simulink model "foc_decoupling_test"  (R2015a)
settings: Solver=ode45  StartTime=0.0  StopTime=0.01  RelTol=1e-3
libraries: simulink x2
settings Model: Creator=user  LastModifiedBy=user

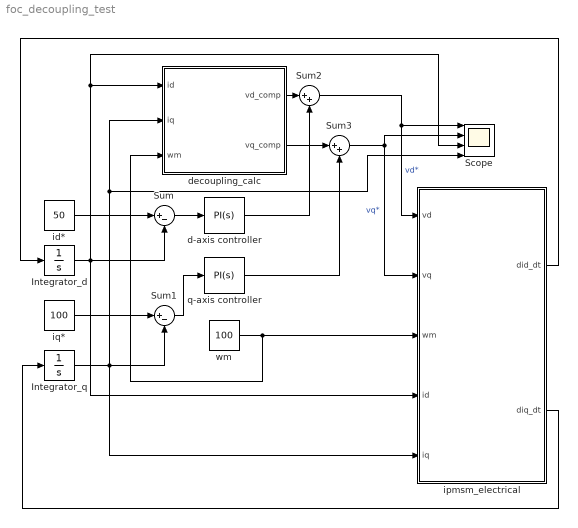
== system foc_decoupling_test ==
  Integrator_d : Integrator
  Integrator_q : Integrator
  Scope : Scope  NumInputPorts=4
      settings: YMin=-5~-5~-5~-5  YMax=5~5~5~5  SaveName=ScopeData2
  Sum : Sum  Inputs=|+-
  Sum1 : Sum  Inputs=|+-
  Sum2 : Sum  Inputs=|++
  Sum3 : Sum  Inputs=|++
  d-axis controller : simulink/Continuous/PID Controller  Controller=PI  TimeDomain=Continuous-time  SampleTime=-1  IntegratorMethod=Forward Euler  FilterMethod=Forward Euler  Form=Parallel  UseFilter=on  ControllerParametersSource=internal  P=0.2827  I=16.6504  D=0  N=100  InitialConditionSource=internal  InitialConditionForIntegrator=0  InitialConditionForFilter=0  ExternalReset=none  LimitOutput=off  UpperSaturationLimit=inf  LowerSaturationLimit=-inf  LinearizeAsGain=on  AntiWindupMode=none  Kb=1  TrackingMode=off  Kt=1  PParamMin=[]  PParamMax=[]  IParamMin=[]  IParamMax=[]  DParamMin=[]  DParamMax=[]  NParamMin=[]  NParamMax=[]  KbParamMin=[]  KbParamMax=[]  KtParamMin=[]  KtParamMax=[]  POutMin=[]  POutMax=[]  IOutMin=[]  IOutMax=[]  DOutMin=[]  DOutMax=[]  NOutMin=[]  NOutMax=[]  KbOutMin=[]  KbOutMax=[]  KtOutMin=[]  KtOutMax=[]  IntegratorOutMin=[]  IntegratorOutMax=[]  FilterOutMin=[]  FilterOutMax=[]  SumOutMin=[]  SumOutMax=[]  SumI1OutMin=[]  SumI1OutMax=[]  SumI2OutMin=[]  SumI2OutMax=[]  SumI3OutMin=[]  SumI3OutMax=[]  SumDOutMin=[]  SumDOutMax=[]  SaturationOutMin=[]  SaturationOutMax=[]  IntegratorContinuousStateAttributes=''  IntegratorStateMustResolveToSignalObject=off  IntegratorRTWStateStorageClass=Auto  FilterContinuousStateAttributes=''  FilterStateMustResolveToSignalObject=off  FilterRTWStateStorageClass=Auto  DifferentiatorICPrevScaledInput=0  DifferentiatorOutMin=[]  DifferentiatorOutMax=[]
  decoupling_calc : MATLAB Function  TreatAsAtomicUnit=on
  id* : Constant  Value=50
  ipmsm_electrical : MATLAB Function  TreatAsAtomicUnit=on
  iq* : Constant  Value=100
  q-axis controller : simulink/Continuous/PID Controller  Controller=PI  TimeDomain=Continuous-time  SampleTime=-1  IntegratorMethod=Forward Euler  FilterMethod=Forward Euler  Form=Parallel  UseFilter=on  ControllerParametersSource=internal  P=0.8011  I=16.6504  D=0  N=100  InitialConditionSource=internal  InitialConditionForIntegrator=0  InitialConditionForFilter=0  ExternalReset=none  LimitOutput=off  UpperSaturationLimit=inf  LowerSaturationLimit=-inf  LinearizeAsGain=on  AntiWindupMode=none  Kb=1  TrackingMode=off  Kt=1  PParamMin=[]  PParamMax=[]  IParamMin=[]  IParamMax=[]  DParamMin=[]  DParamMax=[]  NParamMin=[]  NParamMax=[]  KbParamMin=[]  KbParamMax=[]  KtParamMin=[]  KtParamMax=[]  POutMin=[]  POutMax=[]  IOutMin=[]  IOutMax=[]  DOutMin=[]  DOutMax=[]  NOutMin=[]  NOutMax=[]  KbOutMin=[]  KbOutMax=[]  KtOutMin=[]  KtOutMax=[]  IntegratorOutMin=[]  IntegratorOutMax=[]  FilterOutMin=[]  FilterOutMax=[]  SumOutMin=[]  SumOutMax=[]  SumI1OutMin=[]  SumI1OutMax=[]  SumI2OutMin=[]  SumI2OutMax=[]  SumI3OutMin=[]  SumI3OutMax=[]  SumDOutMin=[]  SumDOutMax=[]  SaturationOutMin=[]  SaturationOutMax=[]  IntegratorContinuousStateAttributes=''  IntegratorStateMustResolveToSignalObject=off  IntegratorRTWStateStorageClass=Auto  FilterContinuousStateAttributes=''  FilterStateMustResolveToSignalObject=off  FilterRTWStateStorageClass=Auto  DifferentiatorICPrevScaledInput=0  DifferentiatorOutMin=[]  DifferentiatorOutMax=[]
  wm : Constant  Value=100
  wires:
  id*/1 -> Sum/1
  Sum/1 -> d-axis controller/1
  iq*/1 -> Sum1/1
  Integrator_q/1 -> decoupling_calc/2(iq), Scope/4, ipmsm_electrical/5(iq), Sum1/2
  Sum1/1 -> q-axis controller/1
  ipmsm_electrical/2(diq_dt) -> Integrator_q/1
  ipmsm_electrical/1(did_dt) -> Integrator_d/1
  Integrator_d/1 -> Scope/3, decoupling_calc/1(id), ipmsm_electrical/4(id), Sum/2
  wm/1 -> decoupling_calc/3(wm), ipmsm_electrical/3(wm)
  decoupling_calc/1(vd_comp) -> Sum2/1
  d-axis controller/1 -> Sum2/2
  decoupling_calc/2(vq_comp) -> Sum3/1
  q-axis controller/1 -> Sum3/2
  Sum3/1 -> Scope/2, ipmsm_electrical/2(vq)  "vq*"
  Sum2/1 -> Scope/1, ipmsm_electrical/1(vd)  "vd*"

== matlab function foc_decoupling_test/decoupling_calc ==
  data: id input; vd_comp output; iq input; wm input; vq_comp output
function [vd_comp, vq_comp] = decoupling_calc(id, iq, wm)
% Feedforward decoupling terms for BMW i3 IPMSM

Ld       = 0.090e-3;
Lq       = 0.255e-3;
lambda_m = 0.0385;
p        = 6;

we = p*wm;

vd_comp = -we*Lq*iq;
vq_comp =  we*(Ld*id + lambda_m);

end

== matlab function foc_decoupling_test/ipmsm_electrical ==
  data: vd input; did_dt output; vq input; wm input; id input; iq input; diq_dt output
function [did_dt, diq_dt] = ipmsm_electrical(vd, vq, wm, id, iq)
% BMW i3 IPMSM dq-axis electrical dynamics
% Units: V, rad/s, A, A/s

Rs       = 5.3e-3;    % Stator resistance, Ohm
Ld       = 0.090e-3;  % d-axis inductance, H
Lq       = 0.255e-3;  % q-axis inductance, H
lambda_m = 0.0385;    % PM flux linkage, Wb
p        = 6;         % Pole pairs

we = p*wm;             % electrical angular velocity, rad/s

did_dt = (vd - Rs*id + we*Lq*iq) / Ld;
diq_dt = (vq - Rs*iq - we*(Ld*id + lambda_m)) / Lq;

end
